simulink model "controller"  (Simulink 8.3)
settings: Solver=FixedStepDiscrete  StartTime=0.0  StopTime=inf  FixedStep=CONFIG.TS  RelTol=1e-3
InitFcn:
  | clc
  | cd(fileparts(which(bdroot)));
  | initTrqBalancingSeeSaw;
values from neighbouring files (symbols this model uses):
  LEFT_RIGHT_FOOT_IN_CONTACT = [1;1]    [initTrqBalancingSeeSaw.m]
undefined symbols (not defined in the file or in its folder): bVectorConstraints, CONFIG, ConstraintsMatrix, directionOfOscillation, gain, noOscillationTime, referenceParams, reg, ROBOT_DOF, sat, seesaw
undefined symbols (not defined in the file): FRAMES
libraries: WBToolboxLibrary x45
settings Model: Creator=makaveli  LastModifiedBy=gabri
settings DataIOCC: SignalLoggingSaveFormat=Dataset
settings DebuggingCC: UnderspecifiedInitializationDetection=Simplified  MergeDetectMultiDrivingBlocksExec=error  FrameProcessingCompatibilityMsg=error  StateNameClashWarn=none
settings GRTTargetCC: CombineOutputUpdateFcns=on  GRTInterface=off
settings ConfigComp: CovMetricSettings=dw  CovHtmlReporting=on  CovSaveCumulativeToWorkspaceVar=on  CovSaveSingleToWorkspaceVar=on  CovExternalEMLEnable=off  CovSFcnEnable=off

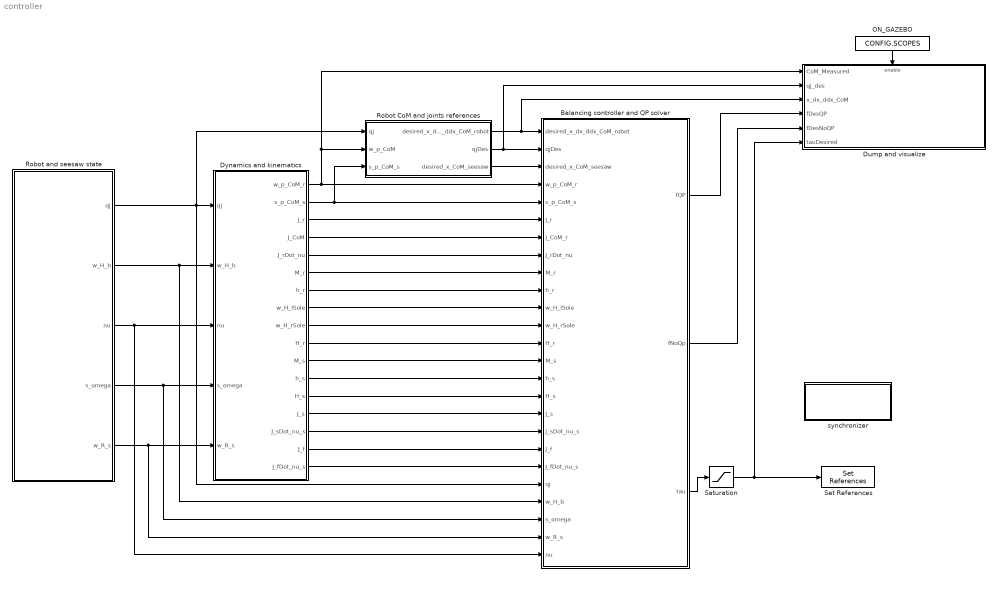
== system controller ==
  Balancing controller and QP solver : Subsystem
  Dump and visualize : Subsystem
  Dynamics and kinematics : Subsystem  Priority=3
  "ON_GAZEBO " : Constant  Value=CONFIG.SCOPES
  Robot CoM and joints references : Subsystem  Priority=2
  Robot and seesaw state : Subsystem
  Saturation : Saturate  UpperLimit=sat.torque  LowerLimit=-sat.torque
  Set References : WBToolboxLibrary/wholeBodyActuators/Set References  controlType=Torque  fullOrSubControl=Full  controlledJoints=''  robotName=WBT_robotName  localName=WBT_modelName  wbiFile=WBT_wbiFilename  wbiList=WBT_wbiList
  synchronizer : Subsystem
      mask Display: disp('SYNCHRONIZER')
  wires:
  Balancing controller and QP solver/1(fQP) -> Dump and visualize/4(fDesQP)
  Balancing controller and QP solver/2(fNoQp) -> Dump and visualize/5(fDesNoQP)
  "ON_GAZEBO "/1 -> Dump and visualize/Enable
  Balancing controller and QP solver/3(tau) -> Saturation/1
  Saturation/1 -> Set References/1, Dump and visualize/6(tauDesired)
  Robot and seesaw state/1(qj) -> Robot CoM and joints references/1(qj), Dynamics and kinematics/1(qj), Balancing controller and QP solver/21(qj)
  Robot and seesaw state/2(w_H_b) -> Dynamics and kinematics/2(w_H_b), Balancing controller and QP solver/22(w_H_b)
  Robot and seesaw state/3(nu) -> Dynamics and kinematics/3(nu), Balancing controller and QP solver/25(nu)
  Robot and seesaw state/4(s_omega) -> Dynamics and kinematics/4(s_omega), Balancing controller and QP solver/23(s_omega)
  Robot and seesaw state/5(w_R_s) -> Dynamics and kinematics/5(w_R_s), Balancing controller and QP solver/24(w_R_s)
  Dynamics and kinematics/2(s_p_CoM_s) -> Robot CoM and joints references/3(s_p_CoM_s), Balancing controller and QP solver/5(s_p_CoM_s)
  Dynamics and kinematics/1(w_p_CoM_r) -> Robot CoM and joints references/2(w_p_CoM), Dump and visualize/1(CoM_Measured), Balancing controller and QP solver/4(w_p_CoM_r)
  Dynamics and kinematics/3(J_r) -> Balancing controller and QP solver/6(J_r)
  Dynamics and kinematics/4(J_CoM) -> Balancing controller and QP solver/7(J_CoM_r)
  Dynamics and kinematics/5(J_rDot_nu) -> Balancing controller and QP solver/8(J_rDot_nu)
  Dynamics and kinematics/6(M_r) -> Balancing controller and QP solver/9(M_r)
  Dynamics and kinematics/7(h_r) -> Balancing controller and QP solver/10(h_r)
  Dynamics and kinematics/8(w_H_lSole) -> Balancing controller and QP solver/11(w_H_lSole)
  Dynamics and kinematics/9(w_H_rSole) -> Balancing controller and QP solver/12(w_H_rSole)
  Dynamics and kinematics/10(H_r) -> Balancing controller and QP solver/13(H_r)
  Dynamics and kinematics/11(M_s) -> Balancing controller and QP solver/14(M_s)
  Dynamics and kinematics/12(h_s) -> Balancing controller and QP solver/15(h_s)
  Dynamics and kinematics/13(H_s) -> Balancing controller and QP solver/16(H_s)
  Dynamics and kinematics/14(J_s) -> Balancing controller and QP solver/17(J_s)
  Robot CoM and joints references/1(desired_x_dx_ddx_CoM_robot) -> Dump and visualize/3(x_dx_ddx_CoM), Balancing controller and QP solver/1(desired_x_dx_ddx_CoM_robot)
  Robot CoM and joints references/3(desired_x_CoM_seesaw) -> Balancing controller and QP solver/3(desired_x_CoM_seesaw)
  Robot CoM and joints references/2(qjDes) -> Dump and visualize/2(qj_des), Balancing controller and QP solver/2(qjDes)
  Dynamics and kinematics/15(J_sDot_nu_s) -> Balancing controller and QP solver/18(J_sDot_nu_s)
  Dynamics and kinematics/16(J_f) -> Balancing controller and QP solver/19(J_f)
  Dynamics and kinematics/17(J_fDot_nu_s) -> Balancing controller and QP solver/20(J_fDot_nu_s)

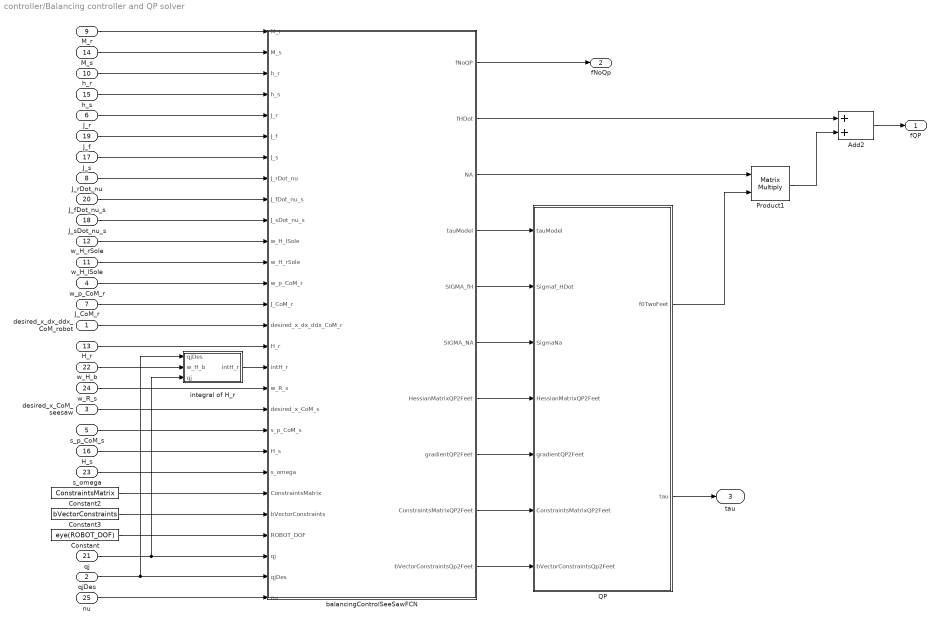
== system controller/Balancing controller and QP solver ==
  desired_x_dx_ddx_CoM_robot : Inport
  qjDes : Inport  Port=2
  desired_x_CoM_seesaw : Inport  Port=3
  w_p_CoM_r : Inport  Port=4
  s_p_CoM_s : Inport  Port=5
  J_r : Inport  Port=6
  J_CoM_r : Inport  Port=7
  J_rDot_nu : Inport  Port=8
  M_r : Inport  Port=9
  h_r : Inport  Port=10
  w_H_lSole : Inport  Port=11
  w_H_rSole : Inport  Port=12
  H_r : Inport  Port=13
  M_s : Inport  Port=14
  h_s : Inport  Port=15
  H_s : Inport  Port=16
  J_s : Inport  Port=17
  J_sDot_nu_s : Inport  Port=18
  J_f : Inport  Port=19
  J_fDot_nu_s : Inport  Port=20
  qj : Inport  Port=21
  w_H_b : Inport  Port=22
  s_omega : Inport  Port=23
  w_R_s : Inport  Port=24
  nu : Inport  Port=25
  "  integral of H_r " : Subsystem
  Add2 : Sum
  Constant : Constant  Value=eye(ROBOT_DOF)
  Constant2 : Constant  Value=ConstraintsMatrix
  Constant3 : Constant  Value=bVectorConstraints
  Product1 : Product  Multiplication=Matrix(*)
  QP : Subsystem
  balancingControlSeeSawFCN : MATLAB Function  TreatAsAtomicUnit=on
  fQP : Outport
  fNoQp : Outport  Port=2
  tau : Outport  Port=3
  wires:
  QP/1(f0TwoFeet) -> Product1/2
  QP/2(tau) -> tau/1
  Product1/1 -> Add2/2
  Add2/1 -> fQP/1
  M_r/1 -> balancingControlSeeSawFCN/1(M_r)
  H_r/1 -> balancingControlSeeSawFCN/16(H_r)
  desired_x_CoM_seesaw/1 -> balancingControlSeeSawFCN/19(desired_x_CoM_s)
  qjDes/1 -> "  integral of H_r "/1(qjDes), balancingControlSeeSawFCN/27(qjDes)
  "  integral of H_r "/1(intH_r) -> balancingControlSeeSawFCN/17(intH_r)
  w_H_b/1 -> "  integral of H_r "/2(w_H_b)
  h_r/1 -> balancingControlSeeSawFCN/3(h_r)
  w_H_rSole/1 -> balancingControlSeeSawFCN/11(w_H_lSole)
  w_H_lSole/1 -> balancingControlSeeSawFCN/12(w_H_rSole)
  J_r/1 -> balancingControlSeeSawFCN/5(J_r)
  J_CoM_r/1 -> balancingControlSeeSawFCN/14(J_CoM_r)
  J_rDot_nu/1 -> balancingControlSeeSawFCN/8(J_rDot_nu)
  w_p_CoM_r/1 -> balancingControlSeeSawFCN/13(w_p_CoM_r)
  s_p_CoM_s/1 -> balancingControlSeeSawFCN/20(s_p_CoM_s)
  desired_x_dx_ddx_CoM_robot/1 -> balancingControlSeeSawFCN/15(desired_x_dx_ddx_CoM_r)
  Constant3/1 -> balancingControlSeeSawFCN/24(bVectorConstraints)
  Constant/1 -> balancingControlSeeSawFCN/25(ROBOT_DOF)
  Constant2/1 -> balancingControlSeeSawFCN/23(ConstraintsMatrix)
  M_s/1 -> balancingControlSeeSawFCN/2(M_s)
  h_s/1 -> balancingControlSeeSawFCN/4(h_s)
  J_f/1 -> balancingControlSeeSawFCN/6(J_f)
  H_s/1 -> balancingControlSeeSawFCN/21(H_s)
  J_sDot_nu_s/1 -> balancingControlSeeSawFCN/10(J_sDot_nu_s)
  J_fDot_nu_s/1 -> balancingControlSeeSawFCN/9(J_fDot_nu_s)
  J_s/1 -> balancingControlSeeSawFCN/7(J_s)
  qj/1 -> "  integral of H_r "/3(qj), balancingControlSeeSawFCN/26(qj)
  s_omega/1 -> balancingControlSeeSawFCN/22(s_omega)
  w_R_s/1 -> balancingControlSeeSawFCN/18(w_R_s)
  balancingControlSeeSawFCN/1(fNoQP) -> fNoQp/1
  balancingControlSeeSawFCN/10(bVectorConstraintsQp2Feet) -> QP/7(bVectorConstraintsQp2Feet)
  balancingControlSeeSawFCN/9(ConstraintsMatrixQP2Feet) -> QP/6(ConstraintsMatrixQP2Feet)
  balancingControlSeeSawFCN/8(gradientQP2Feet) -> QP/5(gradientQP2Feet)
  balancingControlSeeSawFCN/7(HessianMatrixQP2Feet) -> QP/4(HessianMatrixQP2Feet)
  balancingControlSeeSawFCN/6(SIGMA_NA) -> QP/3(SigmaNa)
  balancingControlSeeSawFCN/5(SIGMA_fH) -> QP/2(Sigmaf_HDot)
  balancingControlSeeSawFCN/4(tauModel) -> QP/1(tauModel)
  balancingControlSeeSawFCN/3(NA) -> Product1/1
  balancingControlSeeSawFCN/2(fHDot) -> Add2/1
  nu/1 -> balancingControlSeeSawFCN/28(nu)

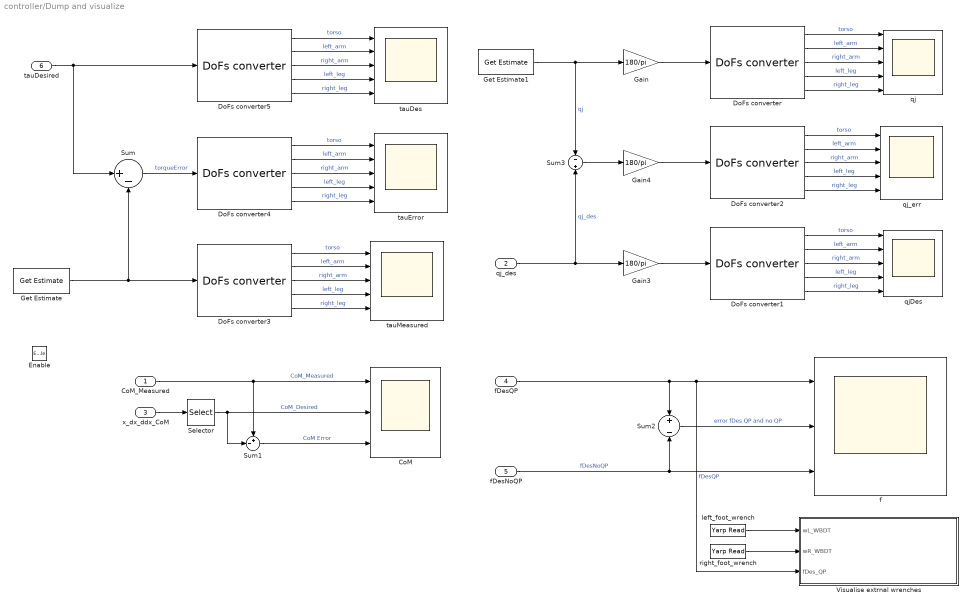
== system controller/Dump and visualize ==
  CoM_Measured : Inport
  qj_des : Inport  Port=2
  x_dx_ddx_CoM : Inport  Port=3
  fDesQP : Inport  Port=4
  fDesNoQP : Inport  Port=5
  tauDesired : Inport  Port=6
  Enable : EnablePort
  CoM : Scope  NumInputPorts=3
  DoFs converter{,1..5} (6 alike) : WBToolboxLibrary/Utilities/DoFs converter  yarp2WBIOption=From WBI to YARP  robotName=WBT_robotName  localName=WBT_modelName  wbiFile=WBT_wbiFilename  wbiList=WBT_wbiList
  Gain : Gain  Gain=180/pi
  Gain3 : Gain  Gain=180/pi
  Gain4 : Gain  Gain=180/pi
  Get Estimate : WBToolboxLibrary/wholeBodyStates/Get Estimate  estimateType=Joints Torque  robotName=WBT_robotName  localName=WBT_modelName  wbiFile=WBT_wbiFilename  wbiList=WBT_wbiList
  Get Estimate1 : WBToolboxLibrary/wholeBodyStates/Get Estimate  estimateType=Joints Position  robotName=WBT_robotName  localName=WBT_modelName  wbiFile=WBT_wbiFilename  wbiList=WBT_wbiList
  Selector : Selector  NumberOfDimensions=2  IndexOptions=Index vector (dialog),Index vector (dialog)  Indices=[1:3],1  OutputSizes=1,1
  Sum : Sum  Inputs=|+-
  Sum1 : Sum  Inputs=+-|
  Sum2 : Sum  Inputs=+|-
  Sum3 : Sum  Inputs=-|+
  "Visualise extrnal wrenches  " : Subsystem
  f : Scope  NumInputPorts=3
  left_foot_wrench : WBToolboxLibrary/Utilities/Yarp Read  portName=PORTS.WBDT_LEFTLEG_EE  signalSize=6  blocking=off  timestamp=off  autoconnect=on  errorOnConnection=on
  qj : Scope  NumInputPorts=5
  qjDes : Scope  NumInputPorts=5
  qj_err : Scope  NumInputPorts=5
  right_foot_wrench : WBToolboxLibrary/Utilities/Yarp Read  portName=PORTS.WBDT_RIGHTLEG_EE  signalSize=6  blocking=off  timestamp=off  autoconnect=on  errorOnConnection=on
  tauDes : Scope  NumInputPorts=5
  tauError : Scope  NumInputPorts=5
  tauMeasured : Scope  NumInputPorts=5
  wires:
  x_dx_ddx_CoM/1 -> Selector/1
  CoM_Measured/1 -> Sum1/1, CoM/1  "CoM_Measured"
  Get Estimate1/1 -> Sum3/1, Gain/1  "qj"
  Gain/1 -> DoFs converter/1
  DoFs converter/5 -> qj/5  "right_leg"
  DoFs converter/1 -> qj/1  "torso"
  DoFs converter/2 -> qj/2  "left_arm"
  DoFs converter/4 -> qj/4  "left_leg"
  DoFs converter/3 -> qj/3  "right_arm"
  fDesQP/1 -> Sum2/1, "Visualise extrnal wrenches  "/3(fDes_QP), f/1  "fDesQP"
  Sum2/1 -> f/2  "error fDes QP and no QP"
  fDesNoQP/1 -> Sum2/2, f/3  "fDesNoQP"
  tauDesired/1 -> DoFs converter5/1, Sum/1
  Get Estimate/1 -> Sum/2, DoFs converter3/1
  DoFs converter5/5 -> tauDes/5  "right_leg"
  DoFs converter5/1 -> tauDes/1  "torso"
  DoFs converter5/2 -> tauDes/2  "left_arm"
  DoFs converter5/4 -> tauDes/4  "left_leg"
  DoFs converter5/3 -> tauDes/3  "right_arm"
  DoFs converter4/5 -> tauError/5  "right_leg"
  DoFs converter4/1 -> tauError/1  "torso"
  DoFs converter4/2 -> tauError/2  "left_arm"
  DoFs converter4/4 -> tauError/4  "left_leg"
  DoFs converter4/3 -> tauError/3  "right_arm"
  Sum/1 -> DoFs converter4/1  "torqueError"
  DoFs converter3/5 -> tauMeasured/5  "right_leg"
  DoFs converter3/1 -> tauMeasured/1  "torso"
  DoFs converter3/2 -> tauMeasured/2  "left_arm"
  DoFs converter3/4 -> tauMeasured/4  "left_leg"
  DoFs converter3/3 -> tauMeasured/3  "right_arm"
  qj_des/1 -> Sum3/2, Gain3/1  "qj_des"
  Gain3/1 -> DoFs converter1/1
  DoFs converter1/5 -> qjDes/5  "right_leg"
  DoFs converter1/1 -> qjDes/1  "torso"
  DoFs converter1/2 -> qjDes/2  "left_arm"
  DoFs converter1/4 -> qjDes/4  "left_leg"
  DoFs converter1/3 -> qjDes/3  "right_arm"
  Gain4/1 -> DoFs converter2/1
  DoFs converter2/5 -> qj_err/5  "right_leg"
  DoFs converter2/1 -> qj_err/1  "torso"
  DoFs converter2/2 -> qj_err/2  "left_arm"
  DoFs converter2/4 -> qj_err/4  "left_leg"
  DoFs converter2/3 -> qj_err/3  "right_arm"
  Sum3/1 -> Gain4/1
  Selector/1 -> Sum1/2, CoM/2  "CoM_Desired"
  Sum1/1 -> CoM/3  "CoM Error"
  right_foot_wrench/1 -> "Visualise extrnal wrenches  "/2(wR_WBDT)
  left_foot_wrench/1 -> "Visualise extrnal wrenches  "/1(wL_WBDT)

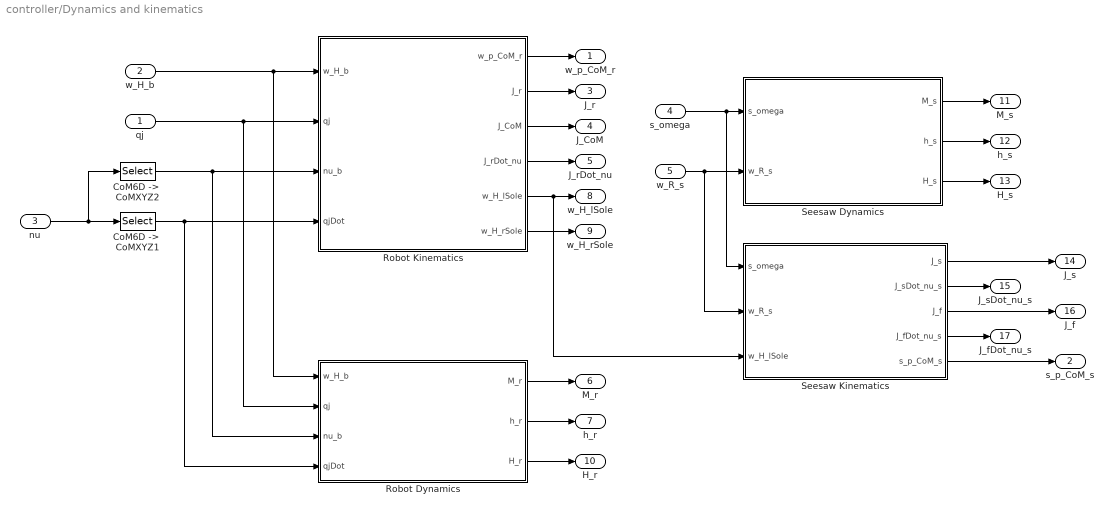
== system controller/Dynamics and kinematics ==
  qj : Inport
  w_H_b : Inport  Port=2
  nu : Inport  Port=3
  s_omega : Inport  Port=4
  w_R_s : Inport  Port=5
  "CoM6D ->  CoMXYZ1" : Selector  InputPortWidth=6+ROBOT_DOF  Indices=[7:6+ROBOT_DOF]
  "CoM6D ->  CoMXYZ2" : Selector  InputPortWidth=6+ROBOT_DOF  Indices=[1 2 3 4 5 6]
  Robot Dynamics : Subsystem
  Robot Kinematics : Subsystem
  Seesaw Dynamics : MATLAB Function  TreatAsAtomicUnit=on
  Seesaw Kinematics : MATLAB Function  TreatAsAtomicUnit=on
  w_p_CoM_r : Outport
  s_p_CoM_s : Outport  Port=2
  J_r : Outport  Port=3
  J_CoM : Outport  Port=4
  J_rDot_nu : Outport  Port=5
  M_r : Outport  Port=6
  h_r : Outport  Port=7
  w_H_lSole : Outport  Port=8
  w_H_rSole : Outport  Port=9
  H_r : Outport  Port=10
  M_s : Outport  Port=11
  h_s : Outport  Port=12
  H_s : Outport  Port=13
  J_s : Outport  Port=14
  J_sDot_nu_s : Outport  Port=15
  J_f : Outport  Port=16
  J_fDot_nu_s : Outport  Port=17
  wires:
  nu/1 -> "CoM6D ->  CoMXYZ1"/1, "CoM6D ->  CoMXYZ2"/1
  Robot Kinematics/1(w_p_CoM_r) -> w_p_CoM_r/1
  Robot Kinematics/2("J_r ") -> J_r/1
  Robot Kinematics/3(J_CoM) -> J_CoM/1
  Robot Kinematics/4(J_rDot_nu) -> J_rDot_nu/1
  Robot Kinematics/5(w_H_lSole) -> Seesaw Kinematics/3(w_H_lSole), w_H_lSole/1
  Robot Kinematics/6(w_H_rSole) -> w_H_rSole/1
  Robot Dynamics/1(M_r) -> M_r/1
  Robot Dynamics/2(h_r) -> h_r/1
  Robot Dynamics/3(H_r) -> H_r/1
  w_H_b/1 -> Robot Dynamics/1(w_H_b), Robot Kinematics/1(w_H_b)
  qj/1 -> Robot Dynamics/2(qj), Robot Kinematics/2(qj)
  "CoM6D ->  CoMXYZ1"/1 -> Robot Dynamics/4(qjDot), Robot Kinematics/4(qjDot)
  "CoM6D ->  CoMXYZ2"/1 -> Robot Dynamics/3(nu_b), Robot Kinematics/3(nu_b)
  w_R_s/1 -> Seesaw Kinematics/2(w_R_s), Seesaw Dynamics/2(w_R_s)
  s_omega/1 -> Seesaw Kinematics/1(s_omega), Seesaw Dynamics/1(s_omega)
  Seesaw Dynamics/3(H_s) -> H_s/1
  Seesaw Dynamics/2(h_s) -> h_s/1
  Seesaw Dynamics/1(M_s) -> M_s/1
  Seesaw Kinematics/1(J_s) -> J_s/1
  Seesaw Kinematics/2(J_sDot_nu_s) -> J_sDot_nu_s/1
  Seesaw Kinematics/3(J_f) -> J_f/1
  Seesaw Kinematics/4(J_fDot_nu_s) -> J_fDot_nu_s/1
  Seesaw Kinematics/5(s_p_CoM_s) -> s_p_CoM_s/1

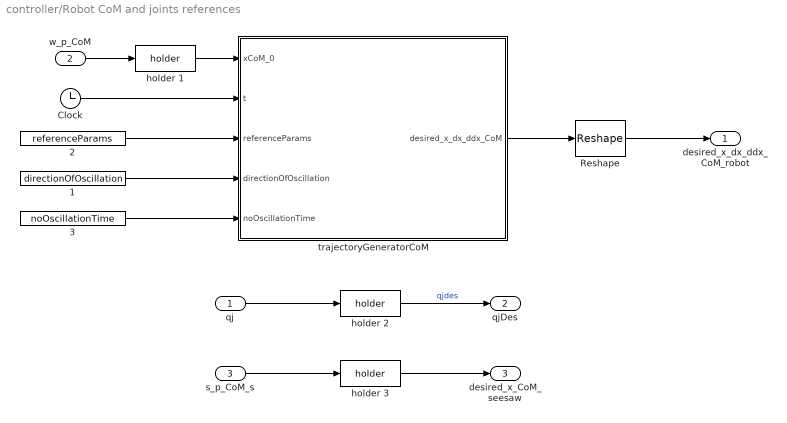
== system controller/Robot CoM and joints references ==
  qj : Inport
  w_p_CoM : Inport  Port=2
  s_p_CoM_s : Inport  Port=3
  "    1" : Constant  Value=directionOfOscillation
  "    2" : Constant  Value=referenceParams
  "    3" : Constant  Value=noOscillationTime
  Clock : Clock
  Reshape : Reshape  OutputDimensionality=Customize  OutputDimensions=[3,3]
  holder 1 : WBToolboxLibrary/Utilities/holder 
  holder 2 : WBToolboxLibrary/Utilities/holder 
  holder 3 : WBToolboxLibrary/Utilities/holder 
  trajectoryGeneratorCoM : MATLAB Function  TreatAsAtomicUnit=on
  desired_x_dx_ddx_CoM_robot : Outport
  qjDes : Outport  Port=2
  desired_x_CoM_seesaw : Outport  Port=3
  wires:
  qj/1 -> holder 2/1
  holder 2/1 -> qjDes/1  "qjdes"
  holder 1/1 -> trajectoryGeneratorCoM/1(xCoM_0)
  "    2"/1 -> trajectoryGeneratorCoM/3(referenceParams)
  Clock/1 -> trajectoryGeneratorCoM/2(t)
  "    1"/1 -> trajectoryGeneratorCoM/4(directionOfOscillation)
  "    3"/1 -> trajectoryGeneratorCoM/5(noOscillationTime)
  trajectoryGeneratorCoM/1(desired_x_dx_ddx_CoM) -> Reshape/1
  Reshape/1 -> desired_x_dx_ddx_CoM_robot/1
  w_p_CoM/1 -> holder 1/1
  holder 3/1 -> desired_x_CoM_seesaw/1
  s_p_CoM_s/1 -> holder 3/1

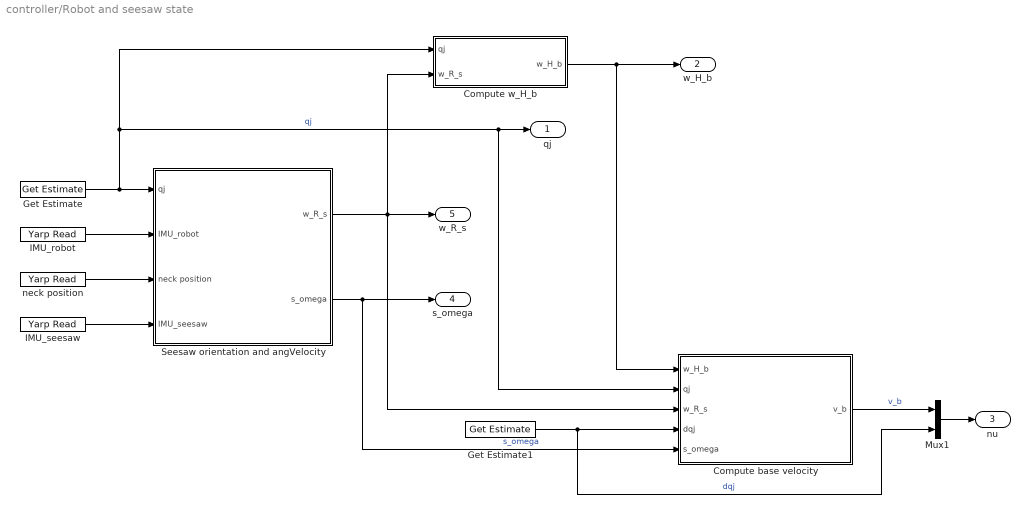
== system controller/Robot and seesaw state ==
  Compute base velocity : Subsystem
  "Compute w_H_b  " : Subsystem
  Get Estimate : WBToolboxLibrary/wholeBodyStates/Get Estimate  estimateType=Joints Position  robotName=WBT_robotName  localName=WBT_modelName  wbiFile=WBT_wbiFilename  wbiList=WBT_wbiList
  Get Estimate1 : WBToolboxLibrary/wholeBodyStates/Get Estimate  estimateType=Joints Velocity  robotName=WBT_robotName  localName=WBT_modelName  wbiFile=WBT_wbiFilename  wbiList=WBT_wbiList
  IMU_robot : WBToolboxLibrary/Utilities/Yarp Read  portName=PORTS.IMU  signalSize=12  blocking=off  timestamp=off  autoconnect=on  errorOnConnection=on
  IMU_seesaw : WBToolboxLibrary/Utilities/Yarp Read  portName=PORTS.IMU_SEESAW  signalSize=12  blocking=off  timestamp=off  autoconnect=on  errorOnConnection=off
  Mux1 : Mux  Inputs=2
  Seesaw orientation and angVelocity : Subsystem
  neck position : WBToolboxLibrary/Utilities/Yarp Read  portName=PORTS.NECK  signalSize=6  blocking=off  timestamp=off  autoconnect=on  errorOnConnection=on
  qj : Outport
  w_H_b : Outport  Port=2
  nu : Outport  Port=3
  s_omega : Outport  Port=4
  w_R_s : Outport  Port=5
  wires:
  IMU_robot/1 -> Seesaw orientation and angVelocity/2(IMU_robot)
  IMU_seesaw/1 -> Seesaw orientation and angVelocity/4(IMU_seesaw)
  neck position/1 -> Seesaw orientation and angVelocity/3(neck position)
  Get Estimate/1 -> "Compute w_H_b  "/1(qj), Compute base velocity/2(qj), qj/1, Seesaw orientation and angVelocity/1(qj)  "qj"
  Mux1/1 -> nu/1
  Compute base velocity/1(v_b) -> Mux1/1  "v_b"
  Seesaw orientation and angVelocity/1(w_R_s) -> w_R_s/1, "Compute w_H_b  "/2(w_R_s), Compute base velocity/3(w_R_s)
  Seesaw orientation and angVelocity/2(s_omega) -> s_omega/1, Compute base velocity/5(s_omega)  "s_omega"
  Get Estimate1/1 -> Mux1/2, Compute base velocity/4(dqj)  "dqj"
  "Compute w_H_b  "/1(w_H_b) -> Compute base velocity/1(w_H_b), w_H_b/1

== system controller/synchronizer ==
  GAZEBO_SYNCHRONIZER : Subsystem
  Logical Operator : Logic  Operator=NOT  AllPortsSameDT=off  OutDataTypeStr=boolean
  "ON_GAZEBO " : Constant  Value=CONFIG.ON_GAZEBO
  REAL_TIME_SYNC : Subsystem
  wires:
  Logical Operator/1 -> REAL_TIME_SYNC/Enable
  "ON_GAZEBO "/1 -> Logical Operator/1, GAZEBO_SYNCHRONIZER/Enable

== system controller/Balancing controller and QP solver/  integral of H_r  ==
  qjDes : Inport
  w_H_b : Inport  Port=2
  qj : Inport  Port=3
  "  " : WBToolboxLibrary/wholeBodyModel/Jacobians/Jacobian  frameName='r_sole'  robotName=WBT_robotName  localName=WBT_modelName  wbiFile=WBT_wbiFilename  wbiList=WBT_wbiList
  Centroidal Momentum : WBToolboxLibrary/wholeBodyModel/Dynamics/Centroidal Momentum  robotName=WBT_robotName  localName=WBT_modelName  wbiFile=WBT_wbiFilename  wbiList=WBT_wbiList
  Constant4 : Constant  Value=LEFT_RIGHT_FOOT_IN_CONTACT
  Jacobian : WBToolboxLibrary/wholeBodyModel/Jacobians/Jacobian  frameName='l_sole'  robotName=WBT_robotName  localName=WBT_modelName  wbiFile=WBT_wbiFilename  wbiList=WBT_wbiList
  MATLAB Function : MATLAB Function  TreatAsAtomicUnit=on
  Sum : Sum  Inputs=|-+
  "holder " : WBToolboxLibrary/Utilities/holder 
  intH_r : Outport
  wires:
  qjDes/1 -> Sum/1, "  "/2, Jacobian/2, Centroidal Momentum/2
  qj/1 -> Sum/2
  Sum/1 -> MATLAB Function/1(qjErr), Centroidal Momentum/4
  MATLAB Function/1(vbEquivalent) -> Centroidal Momentum/3
  Jacobian/1 -> MATLAB Function/2(JL)
  Centroidal Momentum/1 -> intH_r/1
  "  "/1 -> MATLAB Function/3(JR)
  w_H_b/1 -> "holder "/1
  Constant4/1 -> MATLAB Function/4(activeFeetConstraints)
  "holder "/1 -> Centroidal Momentum/1, Jacobian/1, "  "/1

== system controller/Balancing controller and QP solver/QP ==
  tauModel : Inport
  Sigmaf_HDot : Inport  Port=2
  SigmaNa : Inport  Port=3
  HessianMatrixQP2Feet : Inport  Port=4
  gradientQP2Feet : Inport  Port=5
  ConstraintsMatrixQP2Feet : Inport  Port=6
  bVectorConstraintsQp2Feet : Inport  Port=7
  Constant1 : Constant  Value=CONFIG.USE_QP_SOLVER
  Level-2 MATLAB S-Function : M-S-Function  FunctionName=QpBalancingSeesaw
  "ON_GAZEBO " : Constant  Value=CONFIG.SCOPES
  Visualize eventual QP failures : Subsystem
  f0TwoFeet : Outport
  tau : Outport  Port=2
  wires:
  Level-2 MATLAB S-Function/1 -> f0TwoFeet/1
  Level-2 MATLAB S-Function/2 -> Visualize eventual QP failures/1(Exit flag QP two feet)  "Exit flag QP two feet"
  "ON_GAZEBO "/1 -> Visualize eventual QP failures/Enable
  Constant1/1 -> Level-2 MATLAB S-Function/8
  HessianMatrixQP2Feet/1 -> Level-2 MATLAB S-Function/4
  gradientQP2Feet/1 -> Level-2 MATLAB S-Function/5
  ConstraintsMatrixQP2Feet/1 -> Level-2 MATLAB S-Function/6
  bVectorConstraintsQp2Feet/1 -> Level-2 MATLAB S-Function/7
  tauModel/1 -> Level-2 MATLAB S-Function/1
  Sigmaf_HDot/1 -> Level-2 MATLAB S-Function/2
  SigmaNa/1 -> Level-2 MATLAB S-Function/3
  Level-2 MATLAB S-Function/3 -> tau/1

== system controller/Dump and visualize/Visualise extrnal wrenches   ==
  wL_WBDT : Inport
  wR_WBDT : Inport  Port=2
  fDes_QP : Inport  Port=3
  Demux : Demux  Outputs=[6;6]
  Selector : Selector  InputPortWidth=17  Indices=[1:12]
  Sum : Sum  Inputs=-+|
  Sum1 : Sum  Inputs=-+|
  left foot ext wrench : Scope  NumInputPorts=3
  right foot ext wrench : Scope  NumInputPorts=3
  wires:
  wR_WBDT/1 -> right foot ext wrench/1, Sum1/1
  wL_WBDT/1 -> left foot ext wrench/1, Sum/1
  fDes_QP/1 -> Selector/1
  Demux/1 -> Sum/2, left foot ext wrench/2
  Demux/2 -> Sum1/2, right foot ext wrench/2
  Sum/1 -> left foot ext wrench/3
  Sum1/1 -> right foot ext wrench/3
  Selector/1 -> Demux/1

== system controller/Dynamics and kinematics/Robot Dynamics ==
  w_H_b : Inport
  qj : Inport  Port=2
  nu_b : Inport  Port=3
  qjDot : Inport  Port=4
  Centroidal Momentum : WBToolboxLibrary/wholeBodyModel/Dynamics/Centroidal Momentum  robotName=WBT_robotName  localName=WBT_modelName  wbiFile=WBT_wbiFilename  wbiList=WBT_wbiList
  Get Bias Forces : WBToolboxLibrary/wholeBodyModel/Dynamics/Get Bias Forces  robotName=WBT_robotName  localName=WBT_modelName  wbiFile=WBT_wbiFilename  wbiList=WBT_wbiList  explicitGravity=off
  Mass Matrix : WBToolboxLibrary/wholeBodyModel/Dynamics/Mass Matrix  robotName=WBT_robotName  localName=WBT_modelName  wbiFile=WBT_wbiFilename  wbiList=WBT_wbiList
  M_r : Outport
  h_r : Outport  Port=2
  H_r : Outport  Port=3
  wires:
  w_H_b/1 -> Mass Matrix/1, Centroidal Momentum/1, Get Bias Forces/1
  nu_b/1 -> Centroidal Momentum/3, Get Bias Forces/3
  qj/1 -> Centroidal Momentum/2, Get Bias Forces/2, Mass Matrix/2
  qjDot/1 -> Get Bias Forces/4, Centroidal Momentum/4
  Get Bias Forces/1 -> h_r/1
  Centroidal Momentum/1 -> H_r/1
  Mass Matrix/1 -> M_r/1

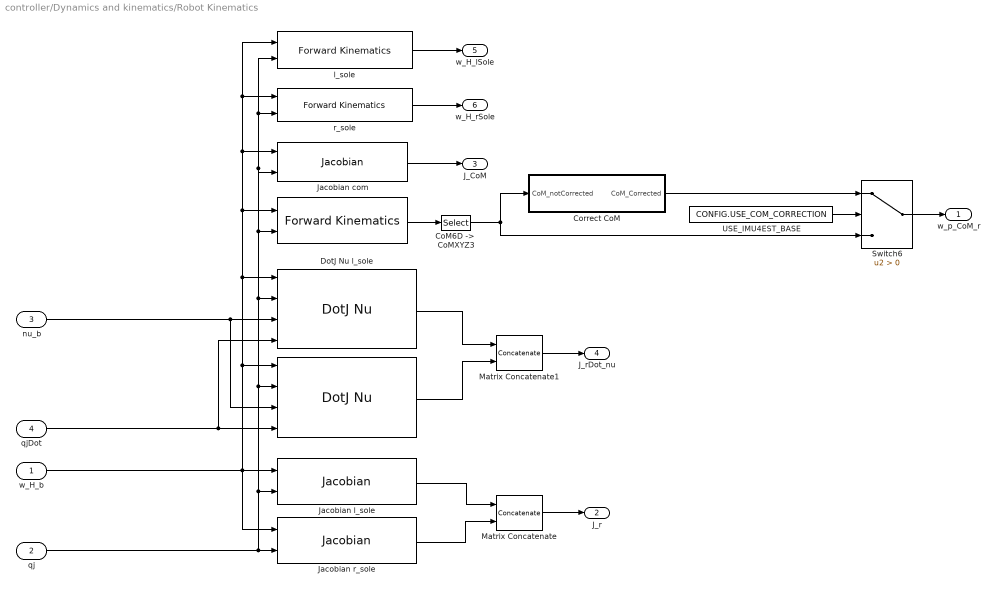
== system controller/Dynamics and kinematics/Robot Kinematics ==
  w_H_b : Inport
  qj : Inport  Port=2
  nu_b : Inport  Port=3
  qjDot : Inport  Port=4
  " " : WBToolboxLibrary/wholeBodyModel/Kinematics/Forward Kinematics  frameName='com'  robotName=WBT_robotName  localName=WBT_modelName  wbiFile=WBT_wbiFilename  wbiList=WBT_wbiList
  "  " : WBToolboxLibrary/wholeBodyModel/Jacobians/DotJ Nu  frameName='r_sole'  robotName=WBT_robotName  localName=WBT_modelName  wbiFile=WBT_wbiFilename  wbiList=WBT_wbiList
  "CoM6D ->  CoMXYZ3" : Selector  NumberOfDimensions=2  InputPortWidth=7  IndexOptions=Index vector (dialog),Index vector (dialog)  Indices=[1 2 3],[4]  OutputSizes=1,1
  Correct CoM : Subsystem
  "DotJ Nu l_sole " : WBToolboxLibrary/wholeBodyModel/Jacobians/DotJ Nu  frameName='l_sole'  robotName=WBT_robotName  localName=WBT_modelName  wbiFile=WBT_wbiFilename  wbiList=WBT_wbiList
  Jacobian com : WBToolboxLibrary/wholeBodyModel/Jacobians/Jacobian  frameName='com'  robotName=WBT_robotName  localName=WBT_modelName  wbiFile=WBT_wbiFilename  wbiList=WBT_wbiList
  Jacobian l_sole : WBToolboxLibrary/wholeBodyModel/Jacobians/Jacobian  frameName='l_sole'  robotName=WBT_robotName  localName=WBT_modelName  wbiFile=WBT_wbiFilename  wbiList=WBT_wbiList
  Jacobian r_sole : WBToolboxLibrary/wholeBodyModel/Jacobians/Jacobian  frameName='r_sole'  robotName=WBT_robotName  localName=WBT_modelName  wbiFile=WBT_wbiFilename  wbiList=WBT_wbiList
  Matrix Concatenate : Concatenate  Mode=Multidimensional array
  Matrix Concatenate1 : Concatenate  Mode=Multidimensional array
  Switch6 : Switch  Criteria=u2 > Threshold
  USE_IMU4EST_BASE : Constant  Value=CONFIG.USE_COM_CORRECTION
  l_sole : WBToolboxLibrary/wholeBodyModel/Kinematics/Forward Kinematics  frameName='l_sole'  robotName=WBT_robotName  localName=WBT_modelName  wbiFile=WBT_wbiFilename  wbiList=WBT_wbiList
  r_sole : WBToolboxLibrary/wholeBodyModel/Kinematics/Forward Kinematics  frameName='r_sole'  robotName=WBT_robotName  localName=WBT_modelName  wbiFile=WBT_wbiFilename  wbiList=WBT_wbiList
  w_p_CoM_r : Outport
  "J_r " : Outport  Port=2
  J_CoM : Outport  Port=3
  J_rDot_nu : Outport  Port=4
  w_H_lSole : Outport  Port=5
  w_H_rSole : Outport  Port=6
  wires:
  qjDot/1 -> "  "/4, "DotJ Nu l_sole "/4
  qj/1 -> r_sole/2, l_sole/2, Jacobian com/2, " "/2, "DotJ Nu l_sole "/2, "  "/2, Jacobian l_sole/2, Jacobian r_sole/2
  nu_b/1 -> "  "/3, "DotJ Nu l_sole "/3
  w_H_b/1 -> "  "/1, r_sole/1, l_sole/1, Jacobian com/1, " "/1, "DotJ Nu l_sole "/1, Jacobian r_sole/1, Jacobian l_sole/1
  Matrix Concatenate1/1 -> J_rDot_nu/1
  Jacobian r_sole/1 -> Matrix Concatenate/2
  l_sole/1 -> w_H_lSole/1
  r_sole/1 -> w_H_rSole/1
  Matrix Concatenate/1 -> "J_r "/1
  Jacobian l_sole/1 -> Matrix Concatenate/1
  Jacobian com/1 -> J_CoM/1
  "DotJ Nu l_sole "/1 -> Matrix Concatenate1/1
  "  "/1 -> Matrix Concatenate1/2
  " "/1 -> "CoM6D ->  CoMXYZ3"/1
  "CoM6D ->  CoMXYZ3"/1 -> Switch6/3, Correct CoM/1(CoM_notCorrected)
  USE_IMU4EST_BASE/1 -> Switch6/2
  Switch6/1 -> w_p_CoM_r/1
  Correct CoM/1(CoM_Corrected) -> Switch6/1

== system controller/Robot and seesaw state/Compute base velocity ==
  w_H_b : Inport
  qj : Inport  Port=2
  w_R_s : Inport  Port=3
  dqj : Inport  Port=4
  s_omega : Inport  Port=5
  Base and joints velocity : Subsystem
  Jacobian fixedLink : WBToolboxLibrary/wholeBodyModel/Jacobians/Jacobian  frameName=FRAMES.fixedLink  robotName=WBT_robotName  localName=WBT_modelName  wbiFile=WBT_wbiFilename  wbiList=WBT_wbiList
  "ON_GAZEBO " : Constant  Value=CONFIG.SCOPES
  evaluateBaseVelocity : MATLAB Function  Priority=10  TreatAsAtomicUnit=on
  v_b : Outport
  wires:
  w_R_s/1 -> evaluateBaseVelocity/2(w_R_s)
  w_H_b/1 -> Jacobian fixedLink/1
  evaluateBaseVelocity/1(v_base) -> Base and joints velocity/1(v_b), v_b/1
  s_omega/1 -> evaluateBaseVelocity/4(s_omega)
  qj/1 -> Jacobian fixedLink/2
  dqj/1 -> evaluateBaseVelocity/3(dqj), Base and joints velocity/2(dqj)
  Jacobian fixedLink/1 -> evaluateBaseVelocity/1(J_fixedLink)
  "ON_GAZEBO "/1 -> Base and joints velocity/Enable

== system controller/Robot and seesaw state/Compute w_H_b   ==
  qj : Inport
  w_R_s : Inport  Port=2
  Compute w_H_fixedLink : Subsystem
  Product1 : Product  Priority=19  Multiplication=Matrix(*)
  fixedLink_H_b : Subsystem  mask{link_name=FRAMES.fixedLink}
      mask prompts: link_name "link name"
      mask help:
      | This block evaluates the homogeneous transformation between the world and the root link, i.e. ^wH_b. It assumes that the link specified by the variable 'link_name' has a constant position
      | w.r.t. an inertial frame, but it can rotate arbitrarily. This rotation is retrived from the IMU sensor.
      mask Display:
      | str = strrep(link_name, '_','\_');
      | port_label('output',1,['{}^{',str '}H_{root}'],'texmode','on')
      | clear str;
      | 
      | port_label('input',1,'q_j','texmode','on')
  w_H_b : Outport
  wires:
  qj/1 -> fixedLink_H_b/1(qj)
  w_R_s/1 -> Compute w_H_fixedLink/1(w_R_s)
  fixedLink_H_b/1(link_H_root) -> Product1/2
  Product1/1 -> w_H_b/1  "w_H_b"
  Compute w_H_fixedLink/1(w_H_fixedLink) -> Product1/1

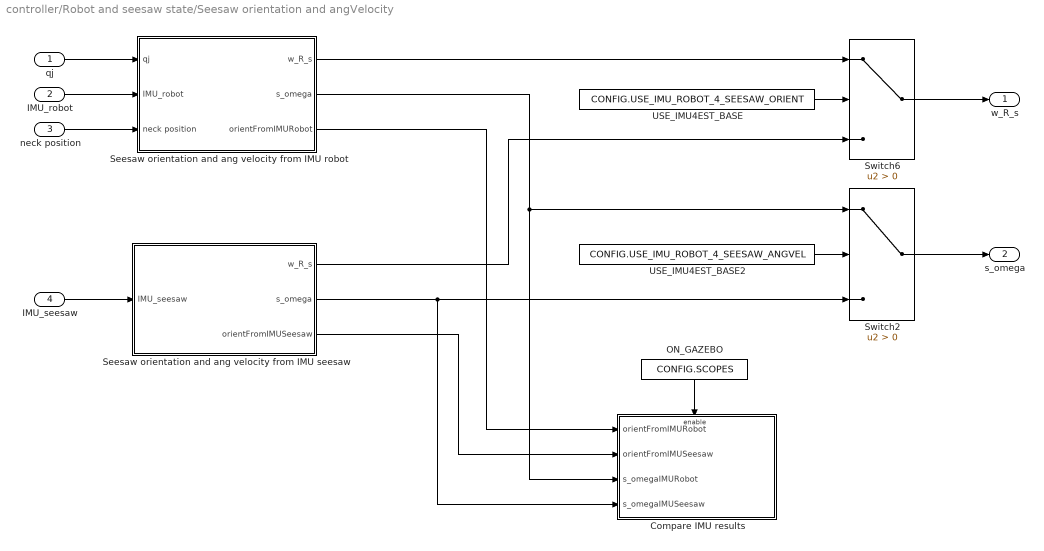
== system controller/Robot and seesaw state/Seesaw orientation and angVelocity ==
  qj : Inport
  IMU_robot : Inport  Port=2
  neck position : Inport  Port=3
  IMU_seesaw : Inport  Port=4
  Compare IMU results : Subsystem
  "ON_GAZEBO " : Constant  Value=CONFIG.SCOPES
  Seesaw orientation and ang velocity from IMU robot : Subsystem
  Seesaw orientation and ang velocity from IMU seesaw : Subsystem
  Switch2 : Switch  Criteria=u2 > Threshold
  Switch6 : Switch  Criteria=u2 > Threshold
  USE_IMU4EST_BASE : Constant  Value=CONFIG.USE_IMU_ROBOT_4_SEESAW_ORIENT
  USE_IMU4EST_BASE2 : Constant  Value=CONFIG.USE_IMU_ROBOT_4_SEESAW_ANGVEL
  w_R_s : Outport
  s_omega : Outport  Port=2
  wires:
  USE_IMU4EST_BASE/1 -> Switch6/2
  Switch6/1 -> w_R_s/1
  Seesaw orientation and ang velocity from IMU seesaw/1(w_R_s) -> Switch6/3
  IMU_seesaw/1 -> Seesaw orientation and ang velocity from IMU seesaw/1(IMU_seesaw)
  Seesaw orientation and ang velocity from IMU robot/1(w_R_s) -> Switch6/1
  neck position/1 -> Seesaw orientation and ang velocity from IMU robot/3(neck position)
  USE_IMU4EST_BASE2/1 -> Switch2/2
  IMU_robot/1 -> Seesaw orientation and ang velocity from IMU robot/2(IMU_robot)
  qj/1 -> Seesaw orientation and ang velocity from IMU robot/1(qj)
  Seesaw orientation and ang velocity from IMU robot/2(s_omega) -> Compare IMU results/3(s_omegaIMURobot), Switch2/1
  Seesaw orientation and ang velocity from IMU seesaw/2(s_omega) -> Compare IMU results/4(s_omegaIMUSeesaw), Switch2/3
  Switch2/1 -> s_omega/1
  Seesaw orientation and ang velocity from IMU robot/3(orientFromIMURobot) -> Compare IMU results/1(orientFromIMURobot)
  Seesaw orientation and ang velocity from IMU seesaw/3(orientFromIMUSeesaw) -> Compare IMU results/2(orientFromIMUSeesaw)
  "ON_GAZEBO "/1 -> Compare IMU results/Enable

== system controller/synchronizer/GAZEBO_SYNCHRONIZER ==
  Enable : EnablePort
  Simulator Synchronizer : WBToolboxLibrary/Utilities/Simulator Synchronizer  period=CONFIG.TS  serverPortName='/clock/rpc'  clientPortName='/WBT_synchronizer/rpc:o'

== system controller/synchronizer/REAL_TIME_SYNC ==
  Enable : EnablePort
  Real Time Synchronizer : WBToolboxLibrary/Utilities/Real Time Synchronizer  period=CONFIG.TS

== system controller/Balancing controller and QP solver/QP/Visualize eventual QP failures ==
  Exit flag QP two feet : Inport
  Enable : EnablePort
  "QP status (0: no failure, 1: not using)" : Scope
  wires:
  Exit flag QP two feet/1 -> "QP status (0: no failure, 1: not using)"/1

== system controller/Dynamics and kinematics/Robot Kinematics/Correct CoM ==
  CoM_notCorrected : Inport
  " " : Constant  Value=0
  "    " : Constant  Value=0
  "CoM6D ->  CoMXYZ4" : Selector  InputPortWidth=3  Indices=[2]
  Mux : Mux  Inputs=3
  Sum : Sum  Inputs=|+-
  "holder " : WBToolboxLibrary/Utilities/holder 
  CoM_Corrected : Outport
  wires:
  CoM_notCorrected/1 -> Sum/1, "CoM6D ->  CoMXYZ4"/1
  Sum/1 -> CoM_Corrected/1
  "CoM6D ->  CoMXYZ4"/1 -> "holder "/1
  " "/1 -> Mux/1
  Mux/1 -> Sum/2
  "holder "/1 -> Mux/2
  "    "/1 -> Mux/3

== system controller/Robot and seesaw state/Compute base velocity/Base and joints velocity ==
  v_b : Inport
  dqj : Inport  Port=2
  Enable : EnablePort
  DoFs converter : WBToolboxLibrary/Utilities/DoFs converter  yarp2WBIOption=From WBI to YARP  robotName=WBT_robotName  localName=WBT_modelName  wbiFile=WBT_wbiFilename  wbiList=WBT_wbiList
  dq_j : Scope  NumInputPorts=5
  vb : Scope
  wires:
  DoFs converter/5 -> dq_j/5  "right_leg"
  DoFs converter/1 -> dq_j/1  "torso"
  DoFs converter/2 -> dq_j/2  "left_arm"
  DoFs converter/4 -> dq_j/4  "left_leg"
  DoFs converter/3 -> dq_j/3  "right_arm"
  dqj/1 -> DoFs converter/1
  v_b/1 -> vb/1

== system controller/Robot and seesaw state/Compute w_H_b  /Compute w_H_fixedLink ==
  w_R_s : Inport
  fixedLink w.r.t the world frame : MATLAB Function  TreatAsAtomicUnit=on
  w_H_fixedLink : Outport
  wires:
  w_R_s/1 -> fixedLink w.r.t the world frame/1(w_R_s)
  fixedLink w.r.t the world frame/1(w_H_fixedLink) -> w_H_fixedLink/1

== system controller/Robot and seesaw state/Compute w_H_b  /fixedLink_H_b ==
  qj : Inport
  Constant2 : Constant  Value=eye(4)
  Constant6 : Constant  Value=eye(4)
  Inv\*1 : Product  Inputs=/*  Multiplication=Matrix(*)
  link : WBToolboxLibrary/wholeBodyModel/Kinematics/Forward Kinematics  frameName=link_name  robotName=WBT_robotName  localName=WBT_modelName  wbiFile=WBT_wbiFilename  wbiList=WBT_wbiList
  root_link : WBToolboxLibrary/wholeBodyModel/Kinematics/Forward Kinematics  frameName='root_link'  robotName=WBT_robotName  localName=WBT_modelName  wbiFile=WBT_wbiFilename  wbiList=WBT_wbiList
  link_H_root : Outport
  wires:
  Constant6/1 -> link/1
  Inv\*1/1 -> link_H_root/1
  link/1 -> Inv\*1/1
  Constant2/1 -> root_link/1
  qj/1 -> root_link/2, link/2
  root_link/1 -> Inv\*1/2

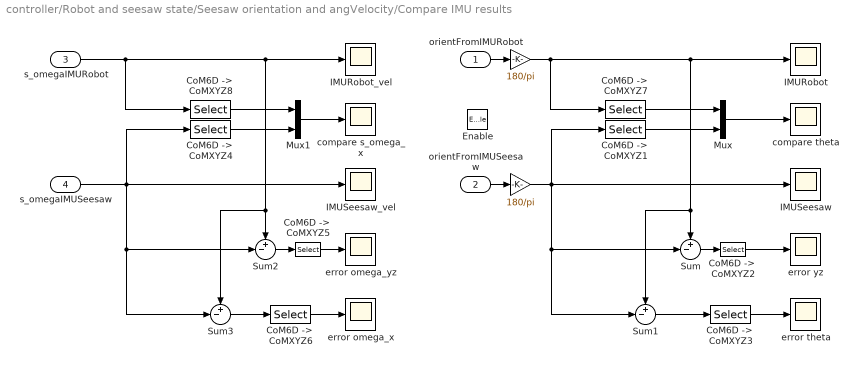
== system controller/Robot and seesaw state/Seesaw orientation and angVelocity/Compare IMU results ==
  orientFromIMURobot : Inport
  orientFromIMUSeesaw : Inport  Port=2
  s_omegaIMURobot : Inport  Port=3
  s_omegaIMUSeesaw : Inport  Port=4
  Enable : EnablePort
  "   " : Gain  Gain=180/pi
  "      " : Gain  Gain=180/pi
  CoM6D ->  CoMXYZ{1,3..4,6..8} (6 alike) : Selector  InputPortWidth=3  Indices=[1]
  "CoM6D ->  CoMXYZ2" : Selector  InputPortWidth=3  Indices=[2 3]
  "CoM6D ->  CoMXYZ5" : Selector  InputPortWidth=3  Indices=[2 3]
  IMURobot : Scope
  IMURobot_vel : Scope
  IMUSeesaw : Scope
  IMUSeesaw_vel : Scope
  Mux : Mux  Inputs=2
  Mux1 : Mux  Inputs=2
  Sum{,1..3} (4 alike) : Sum  Inputs=+-|
  compare s_omega_x : Scope
  compare theta : Scope
  error omega_x : Scope
  error omega_yz : Scope
  error theta : Scope
  error yz : Scope
  wires:
  Mux/1 -> compare theta/1
  Sum1/1 -> "CoM6D ->  CoMXYZ3"/1
  Sum/1 -> "CoM6D ->  CoMXYZ2"/1
  "CoM6D ->  CoMXYZ2"/1 -> error yz/1
  s_omegaIMURobot/1 -> "CoM6D ->  CoMXYZ8"/1, Sum3/1, Sum2/1, IMURobot_vel/1
  s_omegaIMUSeesaw/1 -> Sum2/2, Sum3/2, "CoM6D ->  CoMXYZ4"/1, IMUSeesaw_vel/1
  Mux1/1 -> compare s_omega_x/1
  "CoM6D ->  CoMXYZ4"/1 -> Mux1/2
  "CoM6D ->  CoMXYZ8"/1 -> Mux1/1
  Sum3/1 -> "CoM6D ->  CoMXYZ6"/1
  Sum2/1 -> "CoM6D ->  CoMXYZ5"/1
  "CoM6D ->  CoMXYZ5"/1 -> error omega_yz/1
  "CoM6D ->  CoMXYZ6"/1 -> error omega_x/1
  orientFromIMURobot/1 -> "   "/1
  "CoM6D ->  CoMXYZ1"/1 -> Mux/2
  "CoM6D ->  CoMXYZ7"/1 -> Mux/1
  orientFromIMUSeesaw/1 -> "      "/1
  "CoM6D ->  CoMXYZ3"/1 -> error theta/1
  "   "/1 -> "CoM6D ->  CoMXYZ7"/1, IMURobot/1, Sum1/1, Sum/1
  "      "/1 -> Sum/2, Sum1/2, "CoM6D ->  CoMXYZ1"/1, IMUSeesaw/1

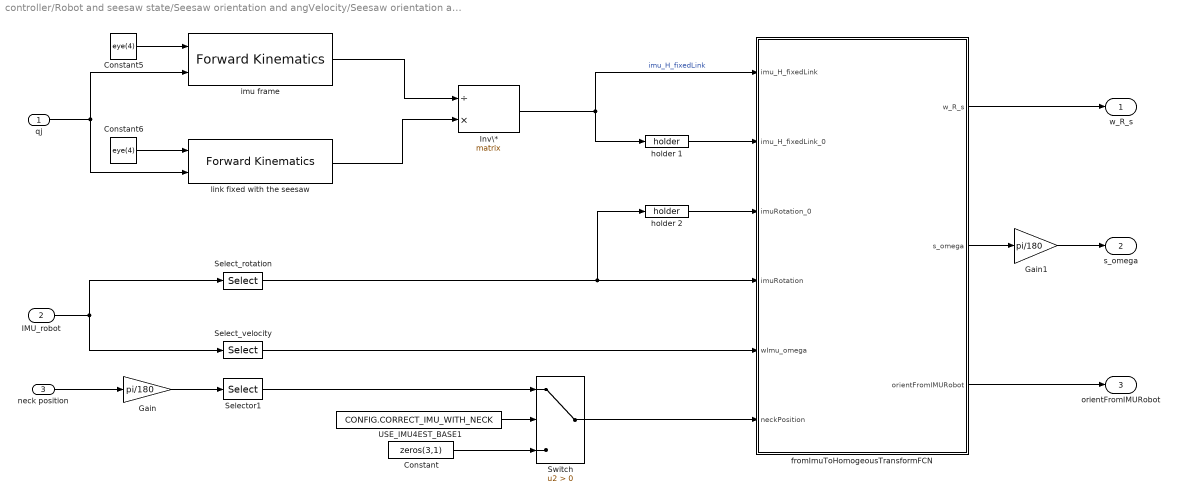
== system controller/Robot and seesaw state/Seesaw orientation and angVelocity/Seesaw orientation and ang velocity from IMU robot ==
  qj : Inport
  IMU_robot : Inport  Port=2
  neck position : Inport  Port=3
  Constant : Constant  Value=zeros(3,1)
  Constant5 : Constant  Value=eye(4)
  Constant6 : Constant  Value=eye(4)
  Gain : Gain  Gain=pi/180
  Gain1 : Gain  Gain=pi/180
  Inv\* : Product  Inputs=/*  Multiplication=Matrix(*)
  Select_rotation : Selector  InputPortWidth=12  Indices=[1 2 3]
  Select_velocity : Selector  InputPortWidth=12  Indices=[7 8 9]
  Selector1 : Selector  InputPortWidth=6  Indices=[1:3]
  Switch : Switch  Criteria=u2 > Threshold
  USE_IMU4EST_BASE1 : Constant  Value=CONFIG.CORRECT_IMU_WITH_NECK
  fromImuToHomogeousTransformFCN : MATLAB Function  TreatAsAtomicUnit=on
  holder 1 : WBToolboxLibrary/Utilities/holder 
  holder 2 : WBToolboxLibrary/Utilities/holder 
  imu frame : WBToolboxLibrary/wholeBodyModel/Kinematics/Forward Kinematics  frameName=FRAMES.imu  robotName=WBT_robotName  localName=WBT_modelName  wbiFile=WBT_wbiFilename  wbiList=WBT_wbiList
  link fixed with the seesaw : WBToolboxLibrary/wholeBodyModel/Kinematics/Forward Kinematics  frameName=FRAMES.fixedLink  robotName=WBT_robotName  localName=WBT_modelName  wbiFile=WBT_wbiFilename  wbiList=WBT_wbiList
  w_R_s : Outport
  s_omega : Outport  Port=2
  orientFromIMURobot : Outport  Port=3
  wires:
  Constant5/1 -> imu frame/1
  Inv\*/1 -> fromImuToHomogeousTransformFCN/1(imu_H_fixedLink), holder 1/1  "imu_H_fixedLink"
  imu frame/1 -> Inv\*/1
  Constant6/1 -> link fixed with the seesaw/1
  link fixed with the seesaw/1 -> Inv\*/2
  qj/1 -> link fixed with the seesaw/2, imu frame/2
  holder 1/1 -> fromImuToHomogeousTransformFCN/2(imu_H_fixedLink_0)
  holder 2/1 -> fromImuToHomogeousTransformFCN/3(imuRotation_0)
  neck position/1 -> Gain/1
  Selector1/1 -> Switch/1
  USE_IMU4EST_BASE1/1 -> Switch/2
  Switch/1 -> fromImuToHomogeousTransformFCN/6(neckPosition)
  Gain/1 -> Selector1/1
  Constant/1 -> Switch/3
  Select_rotation/1 -> fromImuToHomogeousTransformFCN/4(imuRotation), holder 2/1
  IMU_robot/1 -> Select_rotation/1, Select_velocity/1
  Gain1/1 -> s_omega/1
  fromImuToHomogeousTransformFCN/1(w_R_s) -> w_R_s/1
  Select_velocity/1 -> fromImuToHomogeousTransformFCN/5(wImu_omega)
  fromImuToHomogeousTransformFCN/3(orientFromIMURobot) -> orientFromIMURobot/1
  fromImuToHomogeousTransformFCN/2(s_omega) -> Gain1/1

== system controller/Robot and seesaw state/Seesaw orientation and angVelocity/Seesaw orientation and ang velocity from IMU seesaw ==
  IMU_seesaw : Inport
  Gain1 : Gain  Gain=pi/180
  Seesaw angular velocity with IMU seesaw : Subsystem
  Seesaw rotation with IMU_seesaw : Subsystem
  w_R_s : Outport
  s_omega : Outport  Port=2
  orientFromIMUSeesaw : Outport  Port=3
  wires:
  IMU_seesaw/1 -> Seesaw angular velocity with IMU seesaw/1(IMU_seesaw), Seesaw rotation with IMU_seesaw/1(IMU_seesaw)
  Seesaw angular velocity with IMU seesaw/1(s_omega) -> Gain1/1
  Seesaw rotation with IMU_seesaw/1(w_R_s) -> w_R_s/1
  Gain1/1 -> s_omega/1
  Seesaw rotation with IMU_seesaw/2(orientFromIMUSeesaw) -> orientFromIMUSeesaw/1

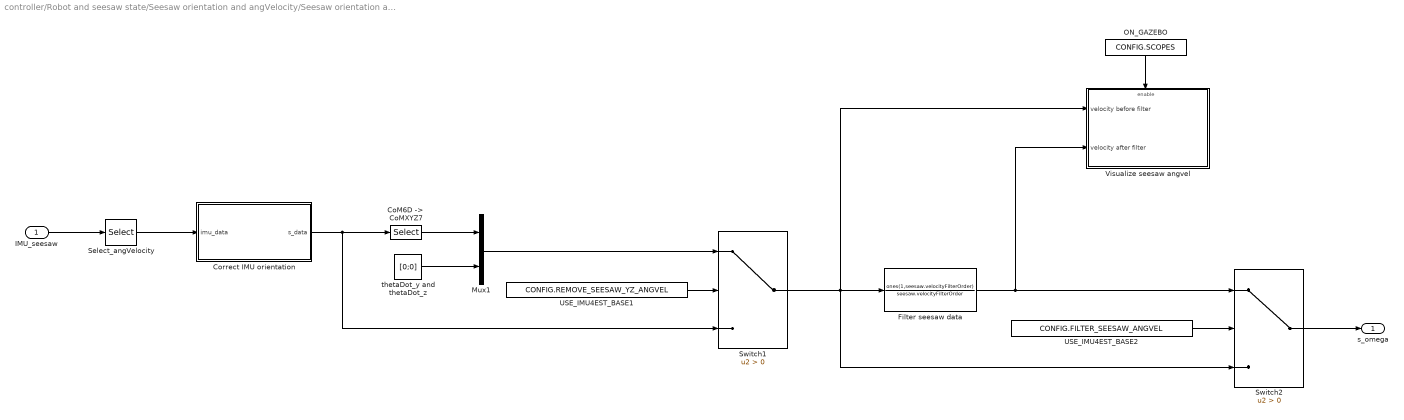
== system controller/Robot and seesaw state/Seesaw orientation and angVelocity/Seesaw orientation and ang velocity from IMU seesaw/Seesaw angular velocity with IMU seesaw ==
  IMU_seesaw : Inport
  "CoM6D ->  CoMXYZ7" : Selector  InputPortWidth=3  Indices=[1]
  Correct IMU orientation : MATLAB Function  TreatAsAtomicUnit=on
  Filter seesaw data : DiscreteFilter  Numerator=ones(1,seesaw.velocityFilterOrder)  Denominator=seesaw.velocityFilterOrder  SampleTime=CONFIG.TS
  Mux1 : Mux  Inputs=2
  "ON_GAZEBO " : Constant  Value=CONFIG.SCOPES
  Select_angVelocity : Selector  InputPortWidth=12  Indices=[7 8 9]
  Switch1 : Switch  Criteria=u2 > Threshold
  Switch2 : Switch  Criteria=u2 > Threshold
  USE_IMU4EST_BASE1 : Constant  Value=CONFIG.REMOVE_SEESAW_YZ_ANGVEL
  USE_IMU4EST_BASE2 : Constant  Value=CONFIG.FILTER_SEESAW_ANGVEL
  Visualize seesaw angvel : Subsystem
  thetaDot_y and thetaDot_z : Constant  Value=[0;0]
  s_omega : Outport
  wires:
  IMU_seesaw/1 -> Select_angVelocity/1
  USE_IMU4EST_BASE1/1 -> Switch1/2
  "CoM6D ->  CoMXYZ7"/1 -> Mux1/1
  thetaDot_y and thetaDot_z/1 -> Mux1/2
  Select_angVelocity/1 -> Correct IMU orientation/1(imu_data)
  Correct IMU orientation/1(s_data) -> "CoM6D ->  CoMXYZ7"/1, Switch1/3
  Mux1/1 -> Switch1/1
  USE_IMU4EST_BASE2/1 -> Switch2/2
  Switch2/1 -> s_omega/1
  Switch1/1 -> Visualize seesaw angvel/1(velocity before filter), Switch2/3, Filter seesaw data/1
  Filter seesaw data/1 -> Switch2/1, Visualize seesaw angvel/2(velocity after filter)
  "ON_GAZEBO "/1 -> Visualize seesaw angvel/Enable

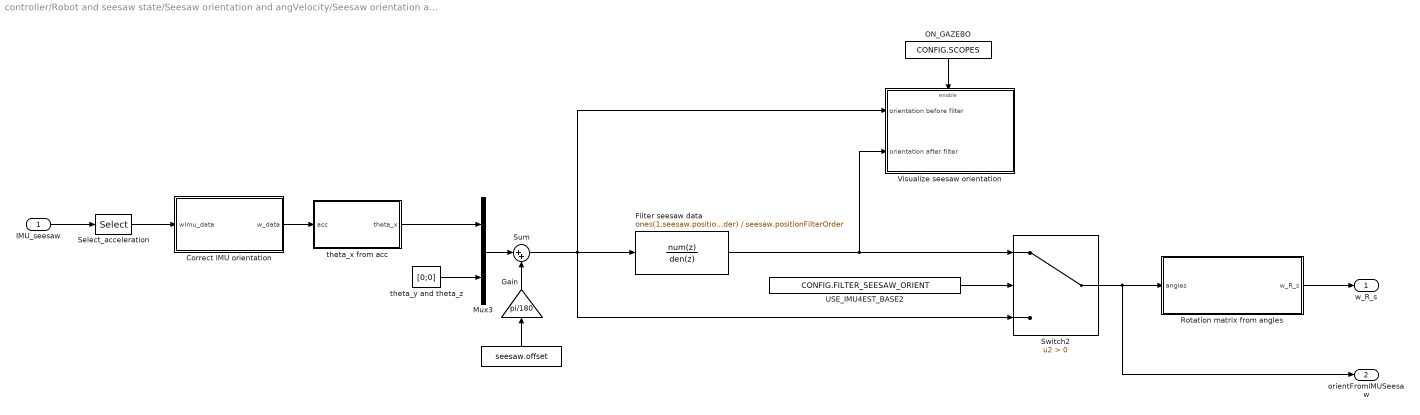
== system controller/Robot and seesaw state/Seesaw orientation and angVelocity/Seesaw orientation and ang velocity from IMU seesaw/Seesaw rotation with IMU_seesaw ==
  IMU_seesaw : Inport
  " " : Constant  Value=seesaw.offset
  Correct IMU orientation : MATLAB Function  TreatAsAtomicUnit=on
  Filter seesaw data : DiscreteFilter  Numerator=ones(1,seesaw.positionFilterOrder)  Denominator=seesaw.positionFilterOrder  SampleTime=CONFIG.TS
  Gain : Gain  Gain=pi/180
  Mux3 : Mux  Inputs=2
  "ON_GAZEBO " : Constant  Value=CONFIG.SCOPES
  Rotation matrix from angles : MATLAB Function  TreatAsAtomicUnit=on
  Select_acceleration : Selector  InputPortWidth=12  Indices=[4 5 6]
  Sum : Sum  Inputs=|++
  Switch2 : Switch  Criteria=u2 > Threshold
  USE_IMU4EST_BASE2 : Constant  Value=CONFIG.FILTER_SEESAW_ORIENT
  Visualize seesaw orientation : Subsystem
  theta_x from acc : MATLAB Function  TreatAsAtomicUnit=on
  theta_y and theta_z : Constant  Value=[0;0]
  w_R_s : Outport
  orientFromIMUSeesaw : Outport  Port=2
  wires:
  theta_x from acc/1(theta_x) -> Mux3/1
  theta_y and theta_z/1 -> Mux3/2
  Correct IMU orientation/1(w_data) -> theta_x from acc/1(acc)
  IMU_seesaw/1 -> Select_acceleration/1
  Select_acceleration/1 -> Correct IMU orientation/1(wImu_data)
  Rotation matrix from angles/1(w_R_s) -> w_R_s/1
  Mux3/1 -> Sum/1
  " "/1 -> Gain/1
  "ON_GAZEBO "/1 -> Visualize seesaw orientation/Enable
  USE_IMU4EST_BASE2/1 -> Switch2/2
  Switch2/1 -> Rotation matrix from angles/1(angles), orientFromIMUSeesaw/1
  Sum/1 -> Switch2/3, Visualize seesaw orientation/1(orientation before filter), Filter seesaw data/1
  Filter seesaw data/1 -> Visualize seesaw orientation/2(orientation after filter), Switch2/1
  Gain/1 -> Sum/2

== system controller/Robot and seesaw state/Seesaw orientation and angVelocity/Seesaw orientation and ang velocity from IMU seesaw/Seesaw angular velocity with IMU seesaw/Visualize seesaw angvel ==
  velocity before filter : Inport
  velocity after filter : Inport  Port=2
  Enable : EnablePort
  Mux : Mux  Inputs=2
  after filter : Scope
  before filter : Scope
  visualize delay : Scope
  wires:
  velocity before filter/1 -> Mux/1, before filter/1
  velocity after filter/1 -> Mux/2, after filter/1
  Mux/1 -> visualize delay/1

== system controller/Robot and seesaw state/Seesaw orientation and angVelocity/Seesaw orientation and ang velocity from IMU seesaw/Seesaw rotation with IMU_seesaw/Visualize seesaw orientation ==
  orientation before filter : Inport
  orientation after filter : Inport  Port=2
  Enable : EnablePort
  Mux : Mux  Inputs=2
  after filter : Scope
  before filter : Scope
  visualize delay : Scope
  wires:
  orientation before filter/1 -> Mux/1, before filter/1
  orientation after filter/1 -> Mux/2, after filter/1
  Mux/1 -> visualize delay/1

== matlab function Balancing controller and QP solver/balancingControlSeeSawFCN ==
  data: fNoQP output double; fHDot output double; NA output double; tauModel output double; SIGMA_fH output double; SIGMA_NA output double; HessianMatrixQP2Feet output double; gradientQP2Feet output double; ConstraintsMatrixQP2Feet output double; bVectorConstraintsQp2Feet output double; M_r input double; M_s input double; h_r input double; h_s input double; J_r input double; J_f input double; J_s input double; J_rDot_nu input double; J_fDot_nu_s input double; J_sDot_nu_s input double; w_H_lSole input double; w_H_rSole input double; w_p_CoM_r input double; J_CoM_r input double; gain parameter double; desired_x_dx_ddx_CoM_r input double; H_r input double; intH_r input double; w_R_s input double; desired_x_CoM_s input double; s_p_CoM_s input double; H_s input double; seesaw parameter double; s_omega input double; reg parameter double; ConstraintsMatrix input double; bVectorConstraints input double; ROBOT_DOF input double; qj input double; qjDes input double; nu input double; CONFIG parameter double
function [fNoQP,fHDot,NA,tauModel,SIGMA_fH,SIGMA_NA,HessianMatrixQP2Feet,gradientQP2Feet,...
          ConstraintsMatrixQP2Feet,bVectorConstraintsQp2Feet] = ...
          ...
          balancingControlFCN(M_r,M_s,h_r,h_s,J_r,J_f,J_s,J_rDot_nu,J_fDot_nu_s,J_sDot_nu_s,w_H_lSole,w_H_rSole,w_p_CoM_r,...
                              J_CoM_r,gain,desired_x_dx_ddx_CoM_r,H_r,intH_r,w_R_s,desired_x_CoM_s,s_p_CoM_s,H_s,seesaw,...
                              s_omega,reg,ConstraintsMatrix,bVectorConstraints,ROBOT_DOF,qj,qjDes,nu,CONFIG)

% Control type 1: control of seesaw and robot momentum toghether
if CONFIG.CONTROL_TYPE == 1
    
         [fNoQP,fHDot,NA,tauModel,SIGMA_fH,SIGMA_NA,HessianMatrixQP2Feet,gradientQP2Feet,...
          ConstraintsMatrixQP2Feet,bVectorConstraintsQp2Feet] = ...
           ...
           balancingControl_v1(M_r,M_s,h_r,h_s,J_r,J_f,J_s,J_rDot_nu,J_fDot_nu_s,J_sDot_nu_s,w_H_lSole,w_H_rSole,w_p_CoM_r,...
                               J_CoM_r,nu,gain,desired_x_dx_ddx_CoM_r,H_r,intH_r,w_R_s,desired_x_CoM_s,s_p_CoM_s,H_s,seesaw,...
                               s_omega,reg,ConstraintsMatrix,bVectorConstraints,ROBOT_DOF,qj,qjDes);
    
else
    
     fNoQP = zeros(17,1);
     fHDot = zeros(17,1);
     NA = zeros(17,17);
     tauModel = zeros(23,1);
     SIGMA_fH = zeros(23,1);
     SIGMA_NA = zeros(23,17);
     HessianMatrixQP2Feet = zeros(17,17);
     gradientQP2Feet = zeros(17,1);
     ConstraintsMatrixQP2Feet = zeros(38,17);
     bVectorConstraintsQp2Feet = zeros(38,1);
                            
end

end

== matlab function Dynamics and kinematics/Seesaw Kinematics ==
  data: J_s output double; s_omega input double; w_R_s input double; w_H_lSole input double; J_sDot_nu_s output double; J_f output double; J_fDot_nu_s output double; seesaw parameter double; s_p_CoM_s output double
function [J_s,J_sDot_nu_s,J_f,J_fDot_nu_s,s_p_CoM_s] = seesawKinematicsFCN(s_omega,w_R_s,w_H_lSole,seesaw)

    [J_s,J_sDot_nu_s,J_f,J_fDot_nu_s,s_p_CoM_s] = seesawKinematics(seesaw,s_omega,w_R_s,w_H_lSole);

end

== matlab function Robot CoM and joints references/trajectoryGeneratorCoM ==
  data: desired_x_dx_ddx_CoM output double; xCoM_0 input double; t input double; referenceParams input double; directionOfOscillation input double; noOscillationTime input double
function desired_x_dx_ddx_CoM = trajectoryGeneratorFCN(xCoM_0, t, referenceParams, directionOfOscillation, noOscillationTime)

desired_x_dx_ddx_CoM = trajectoryGenerator(xCoM_0, t, referenceParams, directionOfOscillation, noOscillationTime);

end

== matlab function Dynamics and kinematics/Seesaw Dynamics ==
  data: M_s output double; s_omega input double; w_R_s input double; h_s output double; H_s output double; seesaw parameter double
function [M_s,h_s,H_s] = seesawDynamicsFCN(s_omega,w_R_s, seesaw)

  [M_s,h_s,H_s] = seesawDynamics(seesaw,s_omega,w_R_s);

end

== matlab function Robot and seesaw state/Seesaw orientation and angVelocity/Seesaw orientation and ang velocity from IMU robot/fromImuToHomogeousTransformFCN ==
  data: imu_H_fixedLink input double; imu_H_fixedLink_0 input double; imuRotation_0 input double; imuRotation input double; wImu_omega input double; neckPosition input double; w_R_s output double; CONFIG parameter double; s_omega output double; orientFromIMURobot output double; seesaw parameter double
function [w_R_s,s_omega,orientFromIMURobot] = fromIMUtoWorldFrameFCN ...
                                              (imu_H_fixedLink,imu_H_fixedLink_0,imuRotation_0,imuRotation,wImu_omega,neckPosition,CONFIG,seesaw)

[w_R_s,s_omega,orientFromIMURobot] = fromIMUtoWorldFrame ...
                                     (imu_H_fixedLink,imu_H_fixedLink_0,imuRotation_0,imuRotation,wImu_omega,neckPosition,CONFIG,seesaw);
 
end

== matlab function Robot and seesaw state/Seesaw orientation and angVelocity/Seesaw orientation and ang velocity from IMU seesaw/Seesaw angular velocity with IMU seesaw/Correct IMU orientation ==
  data: imu_data input double; s_data output double; seesaw parameter double
function s_data = rotateImuWorldFrameFCN(imu_data,seesaw)

% The angular velocity is expressed in a frame attached to the IMU (imu frame), not 
% in wImu frame. Then, this trasformation is giving the angular velocity expressed 
% in the seesaw frame, not in world frame.
s_data = rotateImuWorldFrame(imu_data,seesaw);

end

== matlab function Robot and seesaw state/Seesaw orientation and angVelocity/Seesaw orientation and ang velocity from IMU seesaw/Seesaw rotation with IMU_seesaw/Correct IMU orientation ==
  data: wImu_data input double; w_data output double; seesaw parameter double
function w_data = rotateImuWorldFrameFCN(wImu_data,seesaw)

w_data = rotateImuWorldFrame(wImu_data,seesaw);

end

== matlab function Robot and seesaw state/Seesaw orientation and angVelocity/Seesaw orientation and ang velocity from IMU seesaw/Seesaw rotation with IMU_seesaw/theta_x from acc ==
  data: acc input double; theta_x output double
function theta_x = arctangent(acc)

% theta_x (seesaw roll) in radians
theta_x = atan2(acc(2),acc(3));

end

== matlab function Robot and seesaw state/Seesaw orientation and angVelocity/Seesaw orientation and ang velocity from IMU seesaw/Seesaw rotation with IMU_seesaw/Rotation matrix from angles ==
  data: angles input double; w_R_s output double
function w_R_s = rotationMatrixFromAngles(angles)

% See http://wiki.icub.org/images/8/82/XsensMtx.pdf page 12
w_R_s = rotz(angles(3))*roty(angles(2))*rotx(angles(1));

end

== matlab function Robot and seesaw state/Compute base velocity/evaluateBaseVelocity ==
  data: v_base output double; J_fixedLink input double; w_R_s input double; dqj input double; s_omega input double; seesaw parameter double; reg parameter double
function v_base  = computeBaseVelocityFCN(J_fixedLink,w_R_s,dqj,s_omega,seesaw,reg)

    v_base = computeBaseVelocity(J_fixedLink,w_R_s,dqj,s_omega,seesaw,reg);

end

== matlab function Robot and seesaw state/Compute w_H_b  /Compute w_H_fixedLink/fixedLink w.r.t the world frame ==
  data: w_R_s input double; w_H_fixedLink output double; seesaw parameter double
function w_H_fixedLink = computeTransFromFixedLinkToWorldFCN(w_R_s,seesaw)

w_H_fixedLink = computeTransFromFixedLinkToWorld(w_R_s,seesaw);

end

== matlab function Balancing controller and QP solver/  integral of H_r /MATLAB Function ==
  data: qjErr input double; JL input double; JR input double; vbEquivalent output double; reg parameter double; activeFeetConstraints input double
function vbEquivalent = generateReferencesForH(qjErr,JL,JR,reg,activeFeetConstraints)

% The approximation of integral of angular momentum is given by:
%
%    H_approx = JG(qRef)*(qj-qjDes)
%
% It is assumed here that one of the feet is always on ground at time t=0
% 
if activeFeetConstraints(1) == 1
    
    pinvJb             = (transpose(JL(:,1:6))*JL(:,1:6) + reg.pinvTolVb*eye(6))\transpose(JL(:,1:6));
    vbEquivalent       = -pinvJb*JL(:,7:end)*qjErr;
else
    
    pinvJb             = (transpose(JR(:,1:6))*JR(:,1:6) + reg.pinvTolVb*eye(6))\transpose(JR(:,1:6));
    vbEquivalent       = -pinvJb*JR(:,7:end)*qjErr;
end
end
